simulink model "Controller2"  (R2016a)
settings: Solver=FixedStepAuto  StartTime=0.0  StopTime=inf  FixedStep=0.01  RelTol=1e-3
InitFcn:
  | robotics.ros.createSimulinkBus(gcs);
model workspace (MAT data in the model file):
  SL_ROS_VariableLengthArrays_MaxSizes : struct (value not decoded)
libraries: robotlib x71, simulink x10, dspsrcs4 x6
(part 2 of 2)

== system Controller2/Subsystem/yaw_control/Retrive PID-Parameters ==
  D_yaw : robotlib/Get Parameter  SourceLibraryInfo=This block requires Robotics System Toolbox  ParameterSource=Select from ROS network  ParameterName=/MatlabController/D_yaw  ParameterType=double  ParameterMaxArrayLength=16  ParameterInitialValue=0  SampleTime=-1  ShowErrorCodeOutput=off  ModelName=Controller  BlockId=ParamGet_Controller_937
  I_yaw : robotlib/Get Parameter  SourceLibraryInfo=This block requires Robotics System Toolbox  ParameterSource=Select from ROS network  ParameterName=/MatlabController/I_yaw  ParameterType=double  ParameterMaxArrayLength=16  ParameterInitialValue=0  SampleTime=-1  ShowErrorCodeOutput=off  ModelName=Controller  BlockId=ParamGet_Controller_938
  "N_yaw " : robotlib/Get Parameter  SourceLibraryInfo=This block requires Robotics System Toolbox  ParameterSource=Select from ROS network  ParameterName=/MatlabController/N_yaw  ParameterType=double  ParameterMaxArrayLength=16  ParameterInitialValue=0  SampleTime=-1  ShowErrorCodeOutput=off  ModelName=Controller  BlockId=ParamGet_Controller_939
  P_yaw : robotlib/Get Parameter  SourceLibraryInfo=This block requires Robotics System Toolbox  ParameterSource=Select from ROS network  ParameterName=/MatlabController/P_yaw  ParameterType=double  ParameterMaxArrayLength=16  ParameterInitialValue=0  SampleTime=-1  ShowErrorCodeOutput=off  ModelName=Controller  BlockId=ParamGet_Controller_940
  P : Outport
  I : Outport  Port=2
  D : Outport  Port=3
  N : Outport  Port=4
  wires:
  "N_yaw "/1 -> N/1
  D_yaw/1 -> D/1
  I_yaw/1 -> I/1
  P_yaw/1 -> P/1

== system Controller2/decController/angular_vel x/Retrive PID-Parameters ==
  D_angular_vel_x : robotlib/Get Parameter  SourceLibraryInfo=This block requires Robotics System Toolbox  ParameterSource=Select from ROS network  ParameterName=/matlab_controller/D_angular_vel_x  ParameterType=double  ParameterMaxArrayLength=16  ParameterInitialValue=0  SampleTime=-1  ShowErrorCodeOutput=off  ModelName=Controller  BlockId=ParamGet_Controller_505
  I_angular_vel_x : robotlib/Get Parameter  SourceLibraryInfo=This block requires Robotics System Toolbox  ParameterSource=Select from ROS network  ParameterName=/matlab_controller/I_angular_vel_x  ParameterType=double  ParameterMaxArrayLength=16  ParameterInitialValue=0  SampleTime=-1  ShowErrorCodeOutput=off  ModelName=Controller  BlockId=ParamGet_Controller_506
  "N_angular_vel_x " : robotlib/Get Parameter  SourceLibraryInfo=This block requires Robotics System Toolbox  ParameterSource=Specify your own  ParameterName=/matlab_controller/N_angular_vel_x  ParameterType=double  ParameterMaxArrayLength=16  ParameterInitialValue=0  SampleTime=-1  ShowErrorCodeOutput=off  ModelName=Controller  BlockId=ParamGet_Controller_507
  P_angular_vel_x : robotlib/Get Parameter  SourceLibraryInfo=This block requires Robotics System Toolbox  ParameterSource=Select from ROS network  ParameterName=/matlab_controller/P_angular_vel_x  ParameterType=double  ParameterMaxArrayLength=16  ParameterInitialValue=0  SampleTime=-1  ShowErrorCodeOutput=off  ModelName=Controller  BlockId=ParamGet_Controller_508
  P : Outport
  I : Outport  Port=2
  D : Outport  Port=3
  N : Outport  Port=4
  wires:
  "N_angular_vel_x "/1 -> N/1
  D_angular_vel_x/1 -> D/1
  I_angular_vel_x/1 -> I/1
  P_angular_vel_x/1 -> P/1

== system Controller2/decController/angular_vel y/Retrive PID-Parameters ==
  D_angular_vel_y : robotlib/Get Parameter  SourceLibraryInfo=This block requires Robotics System Toolbox  ParameterSource=Specify your own  ParameterName=/matlab_controller/D_angular_vel_y  ParameterType=double  ParameterMaxArrayLength=16  ParameterInitialValue=0  SampleTime=-1  ShowErrorCodeOutput=off  ModelName=Controller  BlockId=ParamGet_Controller_519
  I_angular_vel_y : robotlib/Get Parameter  SourceLibraryInfo=This block requires Robotics System Toolbox  ParameterSource=Specify your own  ParameterName=/matlab_controller/I_angular_vel_y  ParameterType=double  ParameterMaxArrayLength=16  ParameterInitialValue=0  SampleTime=-1  ShowErrorCodeOutput=off  ModelName=Controller  BlockId=ParamGet_Controller_520
  "N_angular_vel_y " : robotlib/Get Parameter  SourceLibraryInfo=This block requires Robotics System Toolbox  ParameterSource=Specify your own  ParameterName=/matlab_controller/N_angular_vel_y  ParameterType=double  ParameterMaxArrayLength=16  ParameterInitialValue=0  SampleTime=-1  ShowErrorCodeOutput=off  ModelName=Controller  BlockId=ParamGet_Controller_521
  P_angular_vel_y : robotlib/Get Parameter  SourceLibraryInfo=This block requires Robotics System Toolbox  ParameterSource=Specify your own  ParameterName=/matlab_controller/P_angular_vel_y  ParameterType=double  ParameterMaxArrayLength=16  ParameterInitialValue=0  SampleTime=-1  ShowErrorCodeOutput=off  ModelName=Controller  BlockId=ParamGet_Controller_522
  P : Outport
  I : Outport  Port=2
  D : Outport  Port=3
  N : Outport  Port=4
  wires:
  "N_angular_vel_y "/1 -> N/1
  D_angular_vel_y/1 -> D/1
  I_angular_vel_y/1 -> I/1
  P_angular_vel_y/1 -> P/1

== system Controller2/decController/angular_vel z/Retrive PID-Parameters ==
  D_angular_vel_z : robotlib/Get Parameter  SourceLibraryInfo=This block requires Robotics System Toolbox  ParameterSource=Specify your own  ParameterName=/matlab_controller/D_angular_vel_z  ParameterType=double  ParameterMaxArrayLength=16  ParameterInitialValue=0  SampleTime=-1  ShowErrorCodeOutput=off  ModelName=Controller  BlockId=ParamGet_Controller_533
  I_angular_vel_z : robotlib/Get Parameter  SourceLibraryInfo=This block requires Robotics System Toolbox  ParameterSource=Specify your own  ParameterName=/matlab_controller/I_angular_vel_z  ParameterType=double  ParameterMaxArrayLength=16  ParameterInitialValue=0  SampleTime=-1  ShowErrorCodeOutput=off  ModelName=Controller  BlockId=ParamGet_Controller_534
  "N_angular_vel_z " : robotlib/Get Parameter  SourceLibraryInfo=This block requires Robotics System Toolbox  ParameterSource=Specify your own  ParameterName=/matlab_controller/N_angular_vel_z  ParameterType=double  ParameterMaxArrayLength=16  ParameterInitialValue=0  SampleTime=-1  ShowErrorCodeOutput=off  ModelName=Controller  BlockId=ParamGet_Controller_535
  P_angular_vel_z : robotlib/Get Parameter  SourceLibraryInfo=This block requires Robotics System Toolbox  ParameterSource=Specify your own  ParameterName=/matlab_controller/P_angular_vel_z  ParameterType=double  ParameterMaxArrayLength=16  ParameterInitialValue=0  SampleTime=-1  ShowErrorCodeOutput=off  ModelName=Controller  BlockId=ParamGet_Controller_536
  P : Outport
  I : Outport  Port=2
  D : Outport  Port=3
  N : Outport  Port=4
  wires:
  "N_angular_vel_z "/1 -> N/1
  D_angular_vel_z/1 -> D/1
  I_angular_vel_z/1 -> I/1
  P_angular_vel_z/1 -> P/1

== system Controller2/decController/vel x/Retrive PID-Parameters ==
  D_vel_x : robotlib/Get Parameter  SourceLibraryInfo=This block requires Robotics System Toolbox  ParameterSource=Specify your own  ParameterName=/matlab_controller/D_vel_x  ParameterType=double  ParameterMaxArrayLength=16  ParameterInitialValue=0  SampleTime=-1  ShowErrorCodeOutput=off  ModelName=Controller  BlockId=ParamGet_Controller_547
  I_vel_x : robotlib/Get Parameter  SourceLibraryInfo=This block requires Robotics System Toolbox  ParameterSource=Specify your own  ParameterName=/matlab_controller/I_vel_x  ParameterType=double  ParameterMaxArrayLength=16  ParameterInitialValue=0  SampleTime=-1  ShowErrorCodeOutput=off  ModelName=Controller  BlockId=ParamGet_Controller_548
  "N_vel_x " : robotlib/Get Parameter  SourceLibraryInfo=This block requires Robotics System Toolbox  ParameterSource=Specify your own  ParameterName=/matlab_controller/N_vel_x  ParameterType=double  ParameterMaxArrayLength=16  ParameterInitialValue=0  SampleTime=-1  ShowErrorCodeOutput=off  ModelName=Controller  BlockId=ParamGet_Controller_549
  P_vel_x : robotlib/Get Parameter  SourceLibraryInfo=This block requires Robotics System Toolbox  ParameterSource=Specify your own  ParameterName=/matlab_controller/P_vel_x  ParameterType=double  ParameterMaxArrayLength=16  ParameterInitialValue=0  SampleTime=-1  ShowErrorCodeOutput=off  ModelName=Controller  BlockId=ParamGet_Controller_550
  P : Outport
  I : Outport  Port=2
  D : Outport  Port=3
  N : Outport  Port=4
  wires:
  "N_vel_x "/1 -> N/1
  D_vel_x/1 -> D/1
  I_vel_x/1 -> I/1
  P_vel_x/1 -> P/1

== system Controller2/decController/vel y/Retrive PID-Parameters ==
  D_vel_y : robotlib/Get Parameter  SourceLibraryInfo=This block requires Robotics System Toolbox  ParameterSource=Specify your own  ParameterName=/matlab_controller/D_vel_y  ParameterType=double  ParameterMaxArrayLength=16  ParameterInitialValue=0  SampleTime=-1  ShowErrorCodeOutput=off  ModelName=Controller  BlockId=ParamGet_Controller_561
  I_vel_y : robotlib/Get Parameter  SourceLibraryInfo=This block requires Robotics System Toolbox  ParameterSource=Specify your own  ParameterName=/matlab_controller/I_vel_y  ParameterType=double  ParameterMaxArrayLength=16  ParameterInitialValue=0  SampleTime=-1  ShowErrorCodeOutput=off  ModelName=Controller  BlockId=ParamGet_Controller_562
  "N_vel_y " : robotlib/Get Parameter  SourceLibraryInfo=This block requires Robotics System Toolbox  ParameterSource=Specify your own  ParameterName=/matlab_controller/N_vel_y  ParameterType=double  ParameterMaxArrayLength=16  ParameterInitialValue=0  SampleTime=-1  ShowErrorCodeOutput=off  ModelName=Controller  BlockId=ParamGet_Controller_563
  P_vel_y : robotlib/Get Parameter  SourceLibraryInfo=This block requires Robotics System Toolbox  ParameterSource=Specify your own  ParameterName=/matlab_controller/P_vel_y  ParameterType=double  ParameterMaxArrayLength=16  ParameterInitialValue=0  SampleTime=-1  ShowErrorCodeOutput=off  ModelName=Controller  BlockId=ParamGet_Controller_564
  P : Outport
  I : Outport  Port=2
  D : Outport  Port=3
  N : Outport  Port=4
  wires:
  "N_vel_y "/1 -> N/1
  D_vel_y/1 -> D/1
  I_vel_y/1 -> I/1
  P_vel_y/1 -> P/1

== system Controller2/decController/vel z/Retrive PID-Parameters ==
  D_vel_z : robotlib/Get Parameter  SourceLibraryInfo=This block requires Robotics System Toolbox  ParameterSource=Specify your own  ParameterName=/matlab_controller/D_vel_z  ParameterType=double  ParameterMaxArrayLength=16  ParameterInitialValue=0  SampleTime=-1  ShowErrorCodeOutput=off  ModelName=Controller  BlockId=ParamGet_Controller_575
  I_vel_z : robotlib/Get Parameter  SourceLibraryInfo=This block requires Robotics System Toolbox  ParameterSource=Specify your own  ParameterName=/matlab_controller/I_vel_z  ParameterType=double  ParameterMaxArrayLength=16  ParameterInitialValue=0  SampleTime=-1  ShowErrorCodeOutput=off  ModelName=Controller  BlockId=ParamGet_Controller_576
  "N_vel_z " : robotlib/Get Parameter  SourceLibraryInfo=This block requires Robotics System Toolbox  ParameterSource=Specify your own  ParameterName=/matlab_controller/N_vel_z  ParameterType=double  ParameterMaxArrayLength=16  ParameterInitialValue=0  SampleTime=-1  ShowErrorCodeOutput=off  ModelName=Controller  BlockId=ParamGet_Controller_577
  P_vel_z : robotlib/Get Parameter  SourceLibraryInfo=This block requires Robotics System Toolbox  ParameterSource=Specify your own  ParameterName=/matlab_controller/P_vel_z  ParameterType=double  ParameterMaxArrayLength=16  ParameterInitialValue=0  SampleTime=-1  ShowErrorCodeOutput=off  ModelName=Controller  BlockId=ParamGet_Controller_578
  P : Outport
  I : Outport  Port=2
  D : Outport  Port=3
  N : Outport  Port=4
  wires:
  "N_vel_z "/1 -> N/1
  D_vel_z/1 -> D/1
  I_vel_z/1 -> I/1
  P_vel_z/1 -> P/1

== matlab function Controller2/Telegraph/Thruster1 block/MATLAB Function ==
  data: u input; y output; min_scale input; max_scale input
function y = fcn(u,min_scale,max_scale)
%#codegen
    
    if (u < 0)
        y = min_scale*u;
    else
        y = max_scale*u;
    end
end

== matlab function Controller2/thrust alloc1 ==
  data: control_signals input; thrusters output size=6
function thrusters  =...
    thrust_alloc(control_signals)
% lx1 = 0.16;
% ly1 = 0.11;
% ly2 = 0.11;
% lx2 = 0.16;
% ly3 = 0.11;
% lx5 = 0.2;
% ly4 = 0.11;
% lz6 = 0.1; % Måste mätas
% 
% T = [...
%     0, 0, 1, 1, 0, 0;
%     0, 0, 0, 0, 0, -1;
%     -1, -1, 0, 0, -1, 0;
%     ly1, -ly2, 0, 0, 0, lz6;
%     lx1, lx2, 0, 0, -lx5, 0;
%     0, 0, ly3, -ly4, 0, 0];
% 
% T = [...
%         0, 0, 1, 1, 0, 0;
%     0, 0, 0, 0, 0, -1;
%     -1, -1, 0, 0, -1, 0;
%     1, -1, 0, 0, 0, 1;
%     1, 1, 0, 0, -1, 0;
%     0, 0, 1, -1, 0, 0];

% thrust_allocation = (T.')*inv(T*(T.'));

thrust_allocation = [...
         0    0.5000   -0.2500    0.5000    0.2500         0;
         0   -0.5000   -0.2500   -0.5000    0.2500         0;
    0.5000         0         0         0         0    0.5000;
    0.5000         0         0         0         0   -0.5000;
         0         0   -0.5000         0   -0.5000         0;
         0   -1.0000         0         0         0         0];


thrusters = thrust_allocation*control_signals;

end

== matlab function Controller2/states/removeGravity ==
  data: yaw input; pitch input; roll input; x_acc input; y_acc input; z_acc input; x_accnew output; y_accnew output; z_accnew output
function [x_accnew,y_accnew,z_accnew]  = removeGravity(yaw,pitch,roll,x_acc,y_acc,z_acc)
%#codegen

% rotmatrix = [2*w^2+2*x^2-1, 2*x*y-2*w*z, 2*x*z+2*w*y; 
%     2*x*y+2*w*z, 2*w^2+2*y^2-1, 2*x*z-2*w*x;
%     2*x*z-2*w*y, 2*y*z+2*w*x, 2*w^2+2*z^2-1];

sfi = sin(roll);
cfi = cos(roll);
spsi = sin(yaw);
cpsi = cos(yaw);
stheta = sin(pitch);
ctheta = cos(pitch);


rotmatrix = ([...
    cpsi*ctheta, -spsi*cfi+cpsi*stheta*sfi, spsi*sfi+cpsi*cfi*stheta;
    spsi*ctheta, cpsi*cfi+sfi*stheta*spsi, -cpsi*sfi+stheta*spsi*cfi;
    -stheta, ctheta*sfi, ctheta*cfi].');

g = [0;0;9.80];
% Gravity projected in the body fixed frame
acc = rotmatrix*g;

% Removed gravity from the acceleration
x_accnew = x_acc+acc(1);
y_accnew = y_acc+acc(2);
z_accnew = z_acc+acc(3);
end

== matlab function Controller2/toPWM/Calc pwm signal ==
  data: controlsignal input; pwm output
function pwm = calcPWM(controlsignal)
 % thruster values should be between 1100 and 1900 microseconds (us)
 % values less than 1500 us are backwards; values more than are forwards

pwm=(controlsignal + 1) * 400 + 1100;

end

== matlab function Controller2/toPWM/PWM assign ==
  data: blankMessage input Bus: SL_Bus_Controller_std_msgs_UInt16MultiArray; data input size=6; msg output Bus: SL_Bus_Controller_std_msgs_UInt16MultiArray
function msg = assignArray(blankMessage,data)
%#codegen

blankMessage.Data = data;
blankMessage.Layout.DataOffset = uint32(0);
blankMessage.Layout.Dim(1).Stride = uint32(1);
blankMessage.Layout.Dim(1).Size = uint32(6);
blankMessage.Data_SL_Info.CurrentLength = uint32(6);
msg = blankMessage;

end

== stateflow chart Controller2/Telegraph/Thruster1 block/State Transition Table ==
  state state1
  state state2
  (default) -> state1
  state1 -> (junction 20) [order 2]
  (junction 20) -> state1
  state1 -> state2 [order 1] : [x > 0]
      | {u = 1;}
  state2 -> state1 [order 1] : [x> 0]
      | {u= -1;}
  state2 -> (junction 24) [order 2]
  (junction 24) -> state2
  data: x input; u output

== matlab function Controller2/Telegraph/Thruster2 block/MATLAB Function ==
  data: u input; y output; min_scale input; max_scale input
function y = fcn(u,min_scale,max_scale)
%#codegen
    
    if (u < 0)
        y = min_scale*u;
    else
        y = max_scale*u;
    end
end

== stateflow chart Controller2/Telegraph/Thruster2 block/State Transition Table ==
  state state1
  state state2
  (default) -> state1
  state1 -> (junction 20) [order 2]
  (junction 20) -> state1
  state1 -> state2 [order 1] : [x > 0]
      | {u = 1;}
  state2 -> state1 [order 1] : [x> 0]
      | {u= -1;}
  state2 -> (junction 24) [order 2]
  (junction 24) -> state2
  data: x input; u output

== matlab function Controller2/Telegraph/Thruster3 block/MATLAB Function ==
  data: u input; y output; min_scale input; max_scale input
function y = fcn(u,min_scale,max_scale)
%#codegen
    
    if (u < 0)
        y = min_scale*u;
    else
        y = max_scale*u;
    end
end

== stateflow chart Controller2/Telegraph/Thruster3 block/State Transition Table ==
  state state1
  state state2
  (default) -> state1
  state1 -> (junction 20) [order 2]
  (junction 20) -> state1
  state1 -> state2 [order 1] : [x > 0]
      | {u = 1;}
  state2 -> state1 [order 1] : [x> 0]
      | {u= -1;}
  state2 -> (junction 24) [order 2]
  (junction 24) -> state2
  data: x input; u output

== matlab function Controller2/Telegraph/Thruster4 block/MATLAB Function ==
  data: u input; y output; min_scale input; max_scale input
function y = fcn(u,min_scale,max_scale)
%#codegen
    
    if (u < 0)
        y = min_scale*u;
    else
        y = max_scale*u;
    end
end

== stateflow chart Controller2/Telegraph/Thruster4 block/State Transition Table ==
  state state1
  state state2
  (default) -> state1
  state1 -> (junction 20) [order 2]
  (junction 20) -> state1
  state1 -> state2 [order 1] : [x > 0]
      | {u = 1;}
  state2 -> state1 [order 1] : [x> 0]
      | {u= -1;}
  state2 -> (junction 24) [order 2]
  (junction 24) -> state2
  data: x input; u output

== matlab function Controller2/Telegraph/Thruster5 block /MATLAB Function ==
  data: u input; y output; min_scale input; max_scale input
function y = fcn(u,min_scale,max_scale)
%#codegen
    
    if (u < 0)
        y = min_scale*u;
    else
        y = max_scale*u;
    end
end

== stateflow chart Controller2/Telegraph/Thruster5 block /State Transition Table ==
  state state1
  state state2
  (default) -> state1
  state1 -> (junction 20) [order 2]
  (junction 20) -> state1
  state1 -> state2 [order 1] : [x > 0]
      | {u = 1;}
  state2 -> state1 [order 1] : [x> 0]
      | {u= -1;}
  state2 -> (junction 24) [order 2]
  (junction 24) -> state2
  data: x input; u output

== matlab function Controller2/Telegraph/Thruster6 block/MATLAB Function ==
  data: u input; y output; min_scale input; max_scale input
function y = fcn(u,min_scale,max_scale)
%#codegen
    
    if (u < 0)
        y = min_scale*u;
    else
        y = max_scale*u;
    end
end

== stateflow chart Controller2/Telegraph/Thruster6 block/State Transition Table ==
  state state1
  state state2
  (default) -> state1
  state1 -> (junction 20) [order 2]
  (junction 20) -> state1
  state1 -> state2 [order 1] : [x > 0]
      | {u = 1;}
  state2 -> state1 [order 1] : [x> 0]
      | {u= -1;}
  state2 -> (junction 24) [order 2]
  (junction 24) -> state2
  data: x input; u output

== matlab function Controller2/thrust alloc2 ==
  data: control_signals input; thrusters output size=6
function thrusters  =...
    thrust_alloc(control_signals)
% lx1 = 0.16;
% ly1 = 0.11;
% ly2 = 0.11;
% lx2 = 0.16;
% ly3 = 0.11;
% lx5 = 0.2;
% ly4 = 0.11;
% lz6 = 0.1; % Måste mätas
% 
% T = [...
%     0, 0, 1, 1, 0, 0;
%     0, 0, 0, 0, 0, -1;
%     -1, -1, 0, 0, -1, 0;
%     ly1, -ly2, 0, 0, 0, lz6;
%     lx1, lx2, 0, 0, -lx5, 0;
%     0, 0, ly3, -ly4, 0, 0];
% 
% T = [...
%         0, 0, 1, 1, 0, 0;
%     0, 0, 0, 0, 0, -1;
%     -1, -1, 0, 0, -1, 0;
%     1, -1, 0, 0, 0, 1;
%     1, 1, 0, 0, -1, 0;
%     0, 0, 1, -1, 0, 0];

% thrust_allocation = (T.')*inv(T*(T.'));

thrust_allocation = [...
         0    0.5000   -0.2500    0.5000    0.2500         0;
         0   -0.5000   -0.2500   -0.5000    0.2500         0;
    0.5000         0         0         0         0    0.5000;
    0.5000         0         0         0         0   -0.5000;
         0         0   -0.5000         0   -0.5000         0;
         0   -1.0000         0         0         0         0];


thrusters = thrust_allocation*control_signals;

end

== matlab function Controller2/Subsystem/convert to local ==
  data: yaw input; y output size=6; pitch input; roll input; control_vector input
function y = global_to_local(yaw,pitch,roll,control_vector)
%#codegen
sfi = sin(roll);
cfi = cos(roll);
spsi = sin(yaw);
cpsi = cos(yaw);
stheta = sin(pitch);
ctheta = cos(pitch);
r= ([...
    cpsi*ctheta, -spsi*cfi+cpsi*stheta*sfi, spsi*sfi+cpsi*cfi*stheta;
    spsi*ctheta, cpsi*cfi+sfi*stheta*spsi, -cpsi*sfi+stheta*spsi*cfi;
    -stheta, ctheta*sfi, ctheta*cfi]);
rotmatrix = blkdiag(r,r);




y=rotmatrix*control_vector;
end

== matlab function Controller2/thrust alloc ==
  data: control_signals input; thrusters output size=6
function thrusters  =...
    thrust_alloc(control_signals)
% lx1 = 0.16;
% ly1 = 0.11;
% ly2 = 0.11;
% lx2 = 0.16;
% ly3 = 0.11;
% lx5 = 0.2;
% ly4 = 0.11;
% lz6 = 0.1; % Måste mätas
% 
% T = [...
%     0, 0, 1, 1, 0, 0;
%     0, 0, 0, 0, 0, -1;
%     -1, -1, 0, 0, -1, 0;
%     ly1, -ly2, 0, 0, 0, lz6;
%     lx1, lx2, 0, 0, -lx5, 0;
%     0, 0, ly3, -ly4, 0, 0];
% 
% T = [...
%         0, 0, 1, 1, 0, 0;
%     0, 0, 0, 0, 0, -1;
%     -1, -1, 0, 0, -1, 0;
%     1, -1, 0, 0, 0, 1;
%     1, 1, 0, 0, -1, 0;
%     0, 0, 1, -1, 0, 0];

% thrust_allocation = (T.')*inv(T*(T.'));

thrust_allocation = [...
         0    0.5000   -0.2500    0.5000    0.2500         0;
         0   -0.5000   -0.2500   -0.5000    0.2500         0;
    0.5000         0         0         0         0    0.5000;
    0.5000         0         0         0         0   -0.5000;
         0         0   -0.5000         0   -0.5000         0;
         0   -1.0000         0         0         0         0];


thrusters = thrust_allocation*control_signals;

end
